simulink model "battery"  (R2019b)
settings: Solver=VariableStepAuto  StartTime=0.0  StopTime=sim_time  RelTol=1e-3
values from neighbouring files (symbols this model uses):
  Cn = 2.3 * 3600    (= 8280)    [battery_run.m]
  I = 2.3    [battery_run.m]    (also in diff_int.m = 3)
  ocv = Data(:,2)    [battery_run.m]
  R_Charge = Data(:,3)    [battery_run.m]
  R_Discharge = Data(:,4)    [battery_run.m]
  soc = Data(:,1)    [battery_run.m]
settings Model: Creator=dgander  LastModifiedBy=dgander

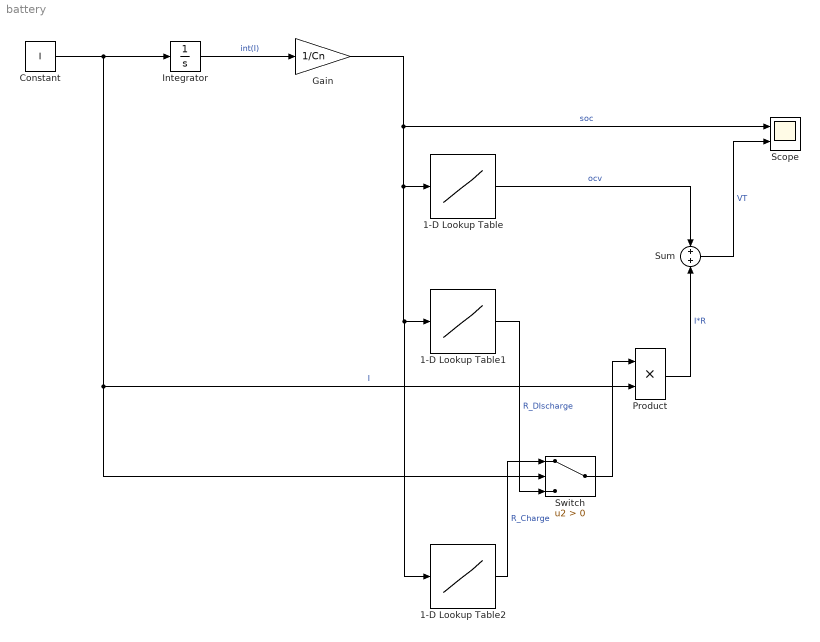
== system battery ==
  1-D Lookup Table : Lookup_n-D  NumberOfTableDimensions=1  BreakpointsForDimension1=soc  Table=R_Discharge  InternalRulePriority=Speed  RndMeth=Simplest  InputSameDT=on
  1-D Lookup Table1 : Lookup_n-D  NumberOfTableDimensions=1  BreakpointsForDimension1=soc  Table=ocv  InternalRulePriority=Speed  RndMeth=Simplest  InputSameDT=on
  1-D Lookup Table2 : Lookup_n-D  NumberOfTableDimensions=1  BreakpointsForDimension1=soc  Table=R_Charge  InternalRulePriority=Speed  RndMeth=Simplest  InputSameDT=on
  Constant : Constant  Value=I
  Gain : Gain  Gain=1/Cn
  Integrator : Integrator
  Product : Product
  Scope : Scope  NumInputPorts=2
  Sum : Sum
  Switch : Switch  Criteria=u2 > Threshold
  wires:
  Constant/1 -> Switch/2, Product/2, Integrator/1  "I"
  Integrator/1 -> Gain/1  "int(I)"
  Gain/1 -> 1-D Lookup Table2/1, 1-D Lookup Table1/1, 1-D Lookup Table/1, Scope/1  "soc"
  1-D Lookup Table/1 -> Sum/1  "ocv"
  1-D Lookup Table1/1 -> Switch/3  "R_DIscharge"
  Product/1 -> Sum/2  "I*R"
  Sum/1 -> Scope/2  "VT"
  1-D Lookup Table2/1 -> Switch/1  "R_Charge"
  Switch/1 -> Product/1
